simulink model "FM_RDS_Receiver_with_RTL_SDR"  (R2020a)
settings: Solver=FixedStepDiscrete  StartTime=0.0  StopTime=inf  RelTol=1e-3  EnableMultiTasking=on
PreLoadFcn:
  | rds_mf_3;
undefined symbols (not defined in the file or in its folder): dfilt, j
libraries: dsparch4 x5, dspobslib x3, dspsrcs4 x2, commutil2 x1, commsrccod2 x1, dspsigops x1, sdrrlib x1
settings Model: Creator=roppel  LastModifiedBy=roppel
settings DataIOCC: LimitDataPoints=on  SaveFormat=Array  ReturnWorkspaceOutputs=off
settings OptimizationCC: LifeSpan=inf
settings DebuggingCC: SolverPrmCheckMsg=warning  SFUnexpectedBacktrackingDiag=warning  SFNoUnconditionalDefaultTransitionDiag=warning  ArithmeticOperatorsInVariantConditions=warning
settings HardwareCC: ProdBitPerPointer=32  ProdBitPerSizeT=32  ProdBitPerPtrDiffT=32  ProdLargestAtomicFloat=None  ProdIntDivRoundTo=Undefined  ProdEndianess=Unspecified  ProdWordSize=32  ProdHWDeviceType=32-bit Generic
settings ModelReferenceCC: PropagateSignalLabelsOutOfModel=off
settings SFSimCC: SimUseLocalCustomCode=off  CustomCodeUndefinedFunction=UseInterfaceOnly
settings RTWCC: RTWUseLocalCustomCode=off
settings CodeAppCC: StateflowObjectComments=on
settings GRTTargetCC: TargetLangStandard=C89/C90 (ANSI)
settings ConfigComp: CovMetricSettings=dw  CovHtmlReporting=on  CovSaveCumulativeToWorkspaceVar=on  CovSaveSingleToWorkspaceVar=on  CovExternalEMLEnable=off  CovSFcnEnable=off

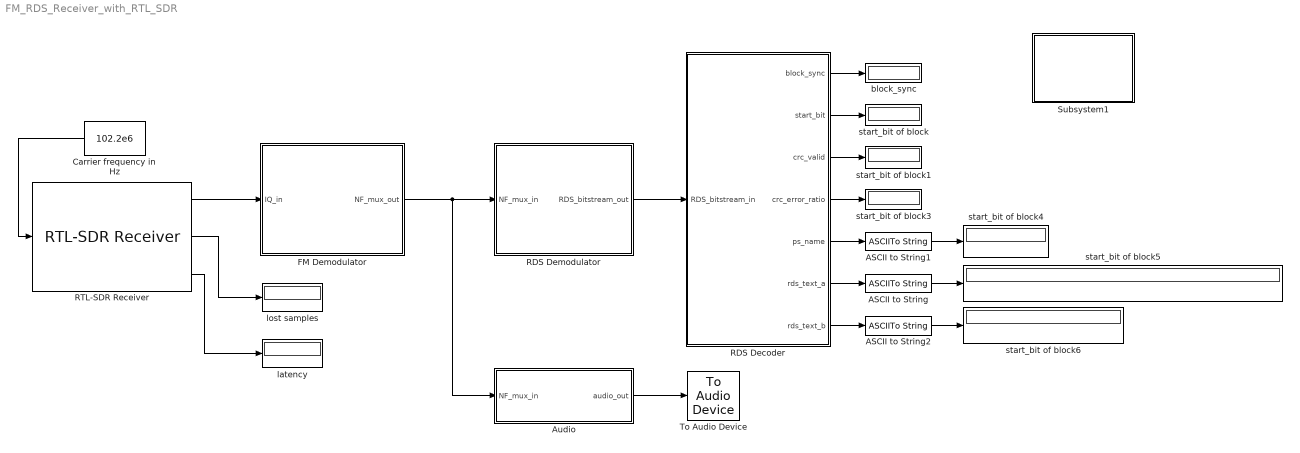
== system FM_RDS_Receiver_with_RTL_SDR ==
  ASCII to String : ASCIIToString
  ASCII to String1 : ASCIIToString
  ASCII to String2 : ASCIIToString
  Audio : Subsystem
  Carrier frequency in Hz : Constant  Value=102.2e6
  FM Demodulator : Subsystem
  RDS Decoder : Subsystem
  RDS Demodulator : Subsystem
  RTL-SDR Receiver : sdrrlib/RTL-SDR Receiver  IPAddress=0  CenterFrequencySource=Input port  CenterFrequency=102.5e6  GainSource=AGC  Gain=50  ADCRate=912e3  FrequencyCorrection=0  LostSamplesOutputPort=on  LatencyOutputPort=on  OutputDataType=single  FrameLength=4864  EnableBurstMode=off  NumFramesInBurst=20  sobjType=sdrr.internal.SDRRTLReceiverSL  dataUDPPort=-1  ctrlUDPPort=-1  subDeviceList=nosubdev  sdrBlockType=SDRBlockTypeSLT.SDRRxBlock  requester=UNUSED_BY_SFCN  sdrExecutionMode=SDRExecutionModeSLT.ExecModeHW  BypassUserLogic=off  DecimatorSelect=DDC decimator  SourceSelect=RF data  SineAmplitude=16000  EnableInternalClock=off  BypassIQBalance=off  IFBandwidth=40e6  ADCRateSource=Dialog  IntermediateFrequency=0  DecimationFactorSource=Dialog  DecimationFactor=512  RFFrequencyIsTunable=logical(1)  SampleTime=(4864)/(912e3)  IFBandwidthSource=Dialog  SineFrequency=30000  BypassDCBlockingFilter=off  IntermediateFrequencySource=Dialog  IQBalanceCoefficients=64  SkipAllHardwareResetAndInitialization=off  EnableIQCalibrationTable=on  CacheIQCalibrationTable=off  EnableOffsetTuning=off  EnableRTLAGC=off  EnableTestMode=off  EnableTunerAGC=on  FrequencyCorrectionSource=Dialog  NumMLBuffers=128  NumUSBBuffers=16  RTLCrystalFrequency=28800000  TunerCrystalFrequency=28800000
      settings: SourceProductBaseCode=RTLSDR
  Subsystem1 : Subsystem  Description=xxx
      settings: OpenFcn=winopen('FM_RDS_Receiver_with_RTL_SDR.pdf')
      mask Display: image('$imagefile'); % Use "Edit Image" on toolstrip to change.
  To Audio Device : dspobslib/To Audio Device  deviceName=Default  inheritSampleRate=on  sampleRate=44100  deviceDatatype=Determine from input data type  autoBufferSize=on  bufferSize=4096  queueDuration=1.0  defaultOutputChannelMapping=on  outputChannelMapping=1  outputNumUnderrunSamples=off
      settings: SourceProductBaseCode=DS
  block_sync : Display
  latency : Display
  lost samples : Display
  start_bit of block{,1,3..6} (6 alike) : Display
  wires:
  RTL-SDR Receiver/1 -> FM Demodulator/1(IQ_in)
  RTL-SDR Receiver/2 -> lost samples/1
  RTL-SDR Receiver/3 -> latency/1
  FM Demodulator/1(NF_mux_out) -> Audio/1(NF_mux_in), RDS Demodulator/1(NF_mux_in)
  Audio/1(audio_out) -> To Audio Device/1
  Carrier frequency in Hz/1 -> RTL-SDR Receiver/1
  RDS Demodulator/1(RDS_bitstream_out) -> RDS Decoder/1(RDS_bitstream_in)
  RDS Decoder/2(start_bit) -> start_bit of block/1
  RDS Decoder/1(block_sync) -> block_sync/1
  RDS Decoder/3(crc_valid) -> start_bit of block1/1
  RDS Decoder/4(crc_error_ratio) -> start_bit of block3/1
  RDS Decoder/6(rds_text_a) -> ASCII to String/1
  ASCII to String/1 -> start_bit of block5/1
  RDS Decoder/5(ps_name) -> ASCII to String1/1
  ASCII to String1/1 -> start_bit of block4/1
  RDS Decoder/7(rds_text_b) -> ASCII to String2/1
  ASCII to String2/1 -> start_bit of block6/1

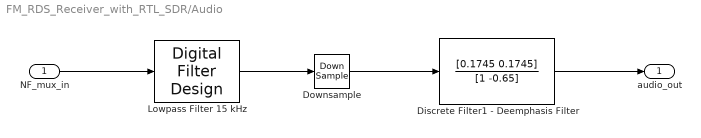
== system FM_RDS_Receiver_with_RTL_SDR/Audio ==
  NF_mux_in : Inport
  Discrete Filter1 - Deemphasis Filter : DiscreteFilter  Numerator=[0.1745 0.1745]  Denominator=[1 -0.65]  InputProcessing=Columns as channels (frame based)  FilterStructure=Direct form I
  Downsample : DownSample  N=19
  Lowpass Filter 15 kHz : dsparch4/Digital Filter Design  mwdsp_browser_bugfix_var=off
  audio_out : Outport
  wires:
  NF_mux_in/1 -> Lowpass Filter 15 kHz/1
  Lowpass Filter 15 kHz/1 -> Downsample/1
  Discrete Filter1 - Deemphasis Filter/1 -> audio_out/1
  Downsample/1 -> Discrete Filter1 - Deemphasis Filter/1

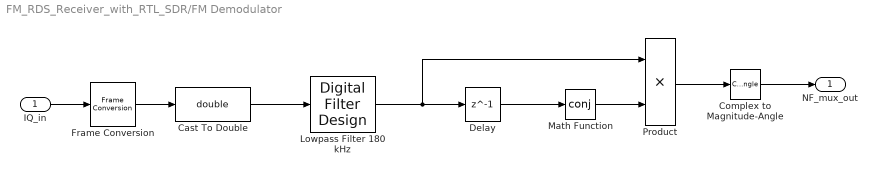
== system FM_RDS_Receiver_with_RTL_SDR/FM Demodulator ==
  IQ_in : Inport
  Cast To Double : DataTypeConversion  OutDataTypeStr=double
  Complex to Magnitude-Angle : ComplexToMagnitudeAngle  Output=Angle
  Delay : Delay  DelayLength=1  InitialCondition=0  InputProcessing=Columns as channels (frame based)
  Frame Conversion : FrameConversion
  Lowpass Filter 180 kHz : dsparch4/Digital Filter Design  mwdsp_browser_bugfix_var=off
  Math Function : Math  Operator=conj  SaturateOnIntegerOverflow=on
  Product : Product
  NF_mux_out : Outport
  wires:
  IQ_in/1 -> Frame Conversion/1
  Product/1 -> Complex to Magnitude-Angle/1
  Math Function/1 -> Product/2
  Delay/1 -> Math Function/1
  Frame Conversion/1 -> Cast To Double/1
  Cast To Double/1 -> Lowpass Filter 180 kHz/1
  Lowpass Filter 180 kHz/1 -> Delay/1, Product/1
  Complex to Magnitude-Angle/1 -> NF_mux_out/1

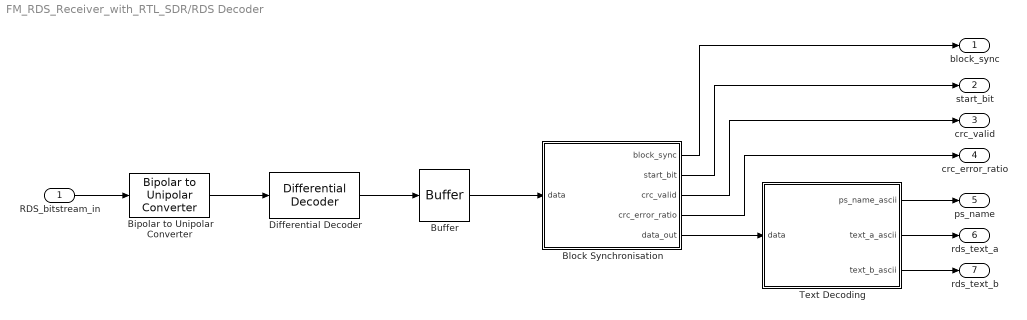
== system FM_RDS_Receiver_with_RTL_SDR/RDS Decoder ==
  RDS_bitstream_in : Inport
  Bipolar to Unipolar Converter : commutil2/Bipolar to Unipolar Converter  M=2  polarity=Positive  dataType=Inherit via internal rule
      settings: SourceProductBaseCode=CM
  Block Synchronisation : MATLAB Function  TreatAsAtomicUnit=on
  Buffer : Buffer  N=10400  V=26
  Differential Decoder : commsrccod2/Differential Decoder  InitCond=0
      settings: SourceProductBaseCode=CM
  Text Decoding : MATLAB Function  TreatAsAtomicUnit=on
  block_sync : Outport
  start_bit : Outport  Port=2
  crc_valid : Outport  Port=3
  crc_error_ratio : Outport  Port=4
  ps_name : Outport  Port=5
  rds_text_a : Outport  Port=6
  rds_text_b : Outport  Port=7
  wires:
  RDS_bitstream_in/1 -> Bipolar to Unipolar Converter/1
  Buffer/1 -> Block Synchronisation/1(data)
  Bipolar to Unipolar Converter/1 -> Differential Decoder/1
  Block Synchronisation/5(data_out) -> Text Decoding/1(data)
  Differential Decoder/1 -> Buffer/1
  Block Synchronisation/1(block_sync) -> block_sync/1
  Block Synchronisation/2(start_bit) -> start_bit/1
  Block Synchronisation/4(crc_error_ratio) -> crc_error_ratio/1
  Text Decoding/1(ps_name_ascii) -> ps_name/1
  Text Decoding/2(text_a_ascii) -> rds_text_a/1
  Text Decoding/3(text_b_ascii) -> rds_text_b/1
  Block Synchronisation/3(crc_valid) -> crc_valid/1

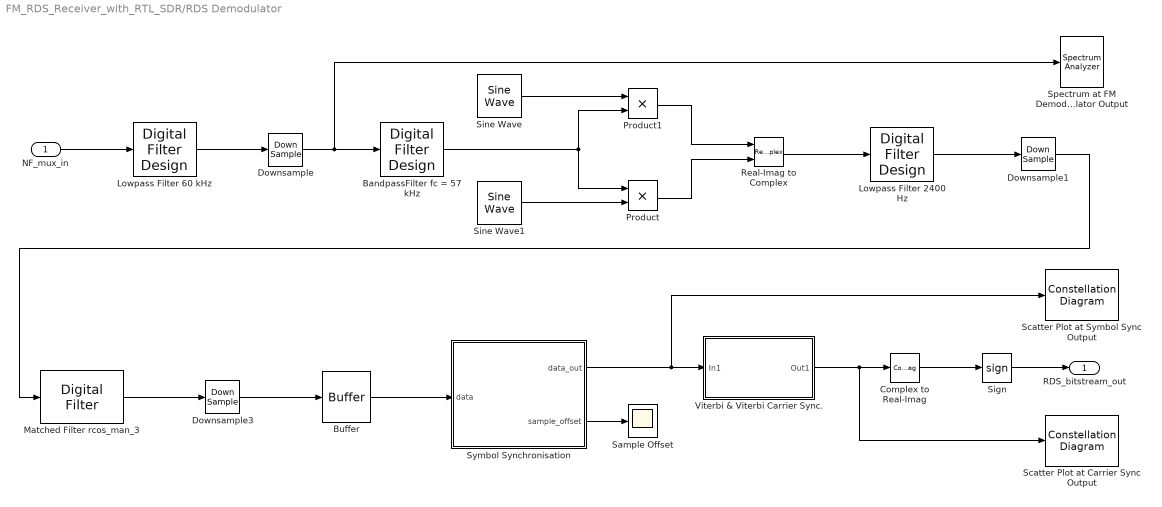
== system FM_RDS_Receiver_with_RTL_SDR/RDS Demodulator ==
  NF_mux_in : Inport
  BandpassFilter fc = 57 kHz : dsparch4/Digital Filter Design  mwdsp_browser_bugfix_var=off
  Buffer : Buffer  N=32*100
  Complex to Real-Imag : ComplexToRealImag  Output=Real
  Downsample : DownSample  N=4  RateOptions=Allow multirate processing
  Downsample1 : DownSample  N=3  RateOptions=Allow multirate processing
  Downsample3 : DownSample  RateOptions=Allow multirate processing
  Lowpass Filter 2400 Hz : dsparch4/Digital Filter Design  mwdsp_browser_bugfix_var=off
  Lowpass Filter 60 kHz : dsparch4/Digital Filter Design  mwdsp_browser_bugfix_var=off
  Matched Filter rcos_man_3 : dspobslib/Digital Filter  TypePopup=FIR (all zeros)  IIRFiltStruct=Direct form II transposed  AllPoleFiltStruct=Direct form  FIRFiltStruct=Direct form  CoeffSource=Specify via dialog  NumCoeffs=rcos_man_3  DenCoeffs=[1 0.1]  BiQuadCoeffs=[1 0.3 0.4 1 0.1 0.2]  LatticeCoeffs=[0.2 0.4]  denIgnore=on  FiltPerSampPopup=One filter per frame  IC=0  ICnum=0  ICden=0  roundingMode=Floor  overflowMode=off  ScaleValues=1  scaleValueFracLength=14  stageInFracLength=15  stageOutFracLength=15  FilterSource=Specify via dialog  dfiltObjectName=dfilt.dffir([1 2 1])  InputProcessing=Columns as channels (frame based)
      settings: SourceProductBaseCode=DS
  Product : Product  RndMeth=Zero  OutDataTypeStr=Inherit: Same as first input
  Product1 : Product  RndMeth=Zero  OutDataTypeStr=Inherit: Same as first input
  Real-Imag to Complex : RealImagToComplex
  Sample Offset : Scope
  Scatter Plot at Carrier Sync Output : ConstellationDiagram
  Scatter Plot at Symbol Sync Output : ConstellationDiagram
  Sign : Signum
  Sine Wave : dspsrcs4/Sine Wave  Amplitude=1  Frequency=57000  Phase=pi/2  SampleMode=Discrete  OutComplex=Real  CompMethod=Table lookup  TableSize=Speed  SampleTime=1/228000  SamplesPerFrame=4864  ResetState=Restart at time zero  OutputFrames=on  dataType=double  wordLen=16  udDataType=sfix(16)  fracBitsMode=Best precision  numFracBits=15  OutDataTypeStr=double  LastOutDataTypeStr=double
  Sine Wave1 : dspsrcs4/Sine Wave  Amplitude=1  Frequency=57000  Phase=-pi  SampleMode=Discrete  OutComplex=Real  CompMethod=Table lookup  TableSize=Speed  SampleTime=1/228000  SamplesPerFrame=4864  ResetState=Restart at time zero  OutputFrames=on  dataType=double  wordLen=16  udDataType=sfix(16)  fracBitsMode=Best precision  numFracBits=15  OutDataTypeStr=double  LastOutDataTypeStr=double
  Spectrum at FM Demodulator Output : SpectrumAnalyzer
  Symbol Synchronisation : MATLAB Function  TreatAsAtomicUnit=on
  Viterbi & Viterbi Carrier Sync. : Subsystem
  RDS_bitstream_out : Outport
  wires:
  Downsample/1 -> BandpassFilter fc = 57 kHz/1, Spectrum at FM Demodulator Output/1
  NF_mux_in/1 -> Lowpass Filter 60 kHz/1
  Lowpass Filter 60 kHz/1 -> Downsample/1
  BandpassFilter fc = 57 kHz/1 -> Product1/2, Product/1
  Sine Wave1/1 -> Product/2
  Product1/1 -> Real-Imag to Complex/1
  Product/1 -> Real-Imag to Complex/2
  Real-Imag to Complex/1 -> Lowpass Filter 2400 Hz/1
  Lowpass Filter 2400 Hz/1 -> Downsample1/1
  Downsample1/1 -> Matched Filter rcos_man_3/1
  Matched Filter rcos_man_3/1 -> Downsample3/1
  Viterbi & Viterbi Carrier Sync./1(Out1) -> Complex to Real-Imag/1, Scatter Plot at Carrier Sync Output/1
  Complex to Real-Imag/1 -> Sign/1
  Sign/1 -> RDS_bitstream_out/1
  Buffer/1 -> Symbol Synchronisation/1(data)
  Downsample3/1 -> Buffer/1
  Sine Wave/1 -> Product1/1
  Symbol Synchronisation/1(data_out) -> Viterbi & Viterbi Carrier Sync./1(In1), Scatter Plot at Symbol Sync Output/1
  Symbol Synchronisation/2(sample_offset) -> Sample Offset/1

== system FM_RDS_Receiver_with_RTL_SDR/Subsystem1 ==

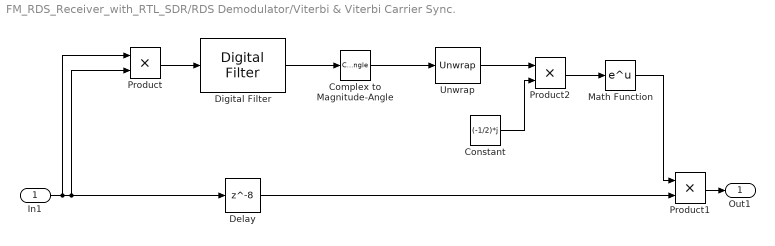
== system FM_RDS_Receiver_with_RTL_SDR/RDS Demodulator/Viterbi & Viterbi Carrier Sync. ==
  In1 : Inport
  Complex to Magnitude-Angle : ComplexToMagnitudeAngle  Output=Angle
  Constant : Constant  Value=(-1/2)*j
  Delay : Delay  DelayLength=8  InitialCondition=0  InputProcessing=Columns as channels (frame based)
  Digital Filter : dspobslib/Digital Filter  TypePopup=FIR (all zeros)  IIRFiltStruct=Direct form II transposed  AllPoleFiltStruct=Direct form  FIRFiltStruct=Direct form  CoeffSource=Specify via dialog  NumCoeffs=ones(1, 17)/17  DenCoeffs=[1 0.1]  BiQuadCoeffs=[1 0.3 0.4 1 0.1 0.2]  LatticeCoeffs=[0.2 0.4]  denIgnore=on  FiltPerSampPopup=One filter per frame  IC=0  ICnum=0  ICden=0  roundingMode=Floor  overflowMode=off  ScaleValues=1  scaleValueFracLength=14  stageInFracLength=15  stageOutFracLength=15  FilterSource=Specify via dialog  dfiltObjectName=dfilt.dffir([1 2 1])  InputProcessing=Columns as channels (frame based)
      settings: SourceProductBaseCode=DS
  Math Function : Math  SignedPower=on  OutputSignalType=complex  SaturateOnIntegerOverflow=on
  Product : Product  RndMeth=Zero
  Product1 : Product  RndMeth=Zero
  Product2 : Product  RndMeth=Zero
  Unwrap : dspsigops/Unwrap  tol=pi  InputProcessing=Columns as channels (frame based)  running=off
  Out1 : Outport
  wires:
  In1/1 -> Product/1, Product/2, Delay/1
  Delay/1 -> Product1/2
  Unwrap/1 -> Product2/1
  Product1/1 -> Out1/1
  Math Function/1 -> Product1/1
  Product/1 -> Digital Filter/1
  Digital Filter/1 -> Complex to Magnitude-Angle/1
  Complex to Magnitude-Angle/1 -> Unwrap/1
  Product2/1 -> Math Function/1
  Constant/1 -> Product2/2

== matlab function FM_RDS_Receiver_with_RTL_SDR/RDS Demodulator/Symbol Synchronisation ==
  data: data_out output; sample_offset output; data input
function [data_out, sample_offset] = fcn(data)
% Carsten Roppel, University of Applied Sciences Schmalkalden
% 02.10.2021

% #codegen

osr = 32;                            % osr samples/bit
nbit = floor(length(data)/osr);      % number of bits
data_out = complex(zeros(nbit, 1));  % output: nbit samples of data
sample_offset = 0;                   % sample offset
max_pwr = 0;                         % maximum power

% downsample data by osr with offset i, calculate power, 
% find offset for maximum power 
for i = 0:(osr-1)
    data_ds = downsample(data, osr, i);
    power = mean(abs(data_ds).^2);
    if power > max_pwr   
        max_pwr = power(1, 1);      
        sample_offset = i;
    end
end

% output: downsampled data using sample_offset
data_ds = downsample(data, osr, sample_offset);
data_ds = data_ds(:, 1);
data_out = data_ds(1:nbit);

end

== matlab function FM_RDS_Receiver_with_RTL_SDR/RDS Decoder/Block Synchronisation ==
  data: block_sync output; start_bit output; crc_valid output; crc_error_ratio output; data input; data_out output
function [block_sync, start_bit, crc_valid, crc_error_ratio, data_out] = fcn(data)
% Carsten Roppel, University of Applied Sciences Schmalkalden
% 02.10.2021

% #codegen

% Requires RDS_offset_word.m

len = 10400;                  % number of bits
nblocks = floor(len/26) - 1;  % number of 26-bit-blocks

% data_out: 399-by-17 matrix
data_out = zeros(nblocks, 17);
block_sync = 0;
next_bit = 1;
start_bit = 1;
offset_word = 0;
crc_errors = 0;
crc_errors_inc = 0;
crc_valid = 0;
crc_error_ratio = 0;

data = data';

while next_bit < len - 25
    % search for valid block
    for i = start_bit:(len-25)
        test = data(i:(i + 25));
        offset_word = RDS_offset_word(test);
        if offset_word ~= 0  % valid block found
            start_bit = i;
            block_sync = 1;
            break;
        else                 % no valid block found
            next_bit = i; 
        end
    end
    
    % extract user data
    if block_sync == 1
        for i = 1:(nblocks - floor(start_bit/26))
            test = data((start_bit + (i - 1)*26):(start_bit + (i - 1)*26 + 25));
            offset_word = RDS_offset_word(test);
            if offset_word == 0
                crc_errors_inc = crc_errors_inc + 1;
                crc_errors = crc_errors + 1;
            else
                crc_errors_inc = 0;
                crc_valid = crc_valid + 1;
            end
            next_bit = start_bit + i*26;
            data_out(i, 1) = offset_word;
            data_out(i, 2:17) = test(1:16);
            % check if 4 consecutive CRC errors
            % if yes, assume loss of sync
            if crc_errors_inc == 4
                block_sync = 0;
                crc_errors_inc = 0;
                start_bit = start_bit + i*26;
                break;
            end
        end
    end
end

crc_error_ratio = crc_errors/(crc_valid + crc_errors);

end

== matlab function FM_RDS_Receiver_with_RTL_SDR/RDS Decoder/Text Decoding ==
  data: data input; ps_name_ascii output; text_a_ascii output; text_b_ascii output
function [ps_name_ascii, text_a_ascii, text_b_ascii] = fcn(data)
% Carsten Roppel, University of Applied Sciences Schmalkalden
% 02.10.2021

% data: 399-by-17 matrix
% Column 1: Block type
%           0: crc_error
%           1: a
%           2: b
%           3: c
%           4: c'
%           5: d
% Columns 2-17: Data bits

btype = data(:, 1);
bdata = data(:, 2:17);
blen = length(bdata);

blockbcount = 0;
% 32 decimal = blank (ASCII)
rds_text_a = zeros(1, 64) + 32;   % Radiotext 64 characters
rds_text_b = zeros(1, 32) + 32;   % Radiotext 32 characters
ps_name = zeros(1, 8) + 32;       % Program Service Name 8 characters

% Search block b
for k = 1:length(btype)
    if btype(k) == 2
        blockbcount = 1;
        % Check group types, see EN50067 Table
        if ~any(xor(bdata(k, (1:5)), [0 0 1 0 0])) 
            % group type 2A -> text in blocks c + d
            % segment address: bits 0 to 3 of block b 
            segment_address = bi2de(flip(bdata(k,(13:16))));
            if (blen >= k + 1 && btype(k+1) == 3)     % check if data contains block c
                char1 = bi2de(flip(bdata(k + 1, (1:8))));
                char2 = bi2de(flip(bdata(k + 1, (9:16))));
                if char1 == 0
                    char1 = 32;
                elseif char2 == 0
                    char2 = 32;
                end                
                rds_text_a(4*segment_address + 1) = char1;
                rds_text_a(4*segment_address + 2) = char2;
            end
            
            if (blen >= k + 2 && btype(k+2) == 5)     % check if data contains block d
                char1 = bi2de(flip(bdata(k + 2, (1:8))));
                char2 = bi2de(flip(bdata(k + 2, (9:16))));
                if char1 == 0
                    char1 = 32;
                elseif char2 == 0
                    char2 = 32;
                end                
                rds_text_a(4*segment_address + 3) = char1;
                rds_text_a(4*segment_address + 4) = char2;
            end
            
        elseif ~any(xor(bdata(k,(1:5)), [0 0 1 0 1]))
            % group type 2B -> text in block d 
            % segment address: bits 0 to 3 of block b 
            segment_address = bi2de(flip(bdata(k,(13:16)))); 
            if (blen >= k + 2 && btype(k+2) == 5)     % check if data contains block d
                char1 = bi2de(flip(bdata(k + 2, (1:8))));
                char2 = bi2de(flip(bdata(k + 2, (9:16))));
                if char1 == 0
                    char1 = 32;
                elseif char2 == 0
                    char2 = 32;
                end                
                rds_text_b(2*segment_address + 1) = char1;
                rds_text_b(2*segment_address + 2) = char2;
            end
            
        elseif ~any(xor(bdata(k,(1:5)), [0 0 0 0 0]))
            % group type = 0A -> ps name in block d
            % segment address: bits 0 to 1 of block b 
            segment_address = bi2de(flip(bdata(k,(15:16))));            
            if (blen >= k + 2 && btype(k+2) == 5)     % check if data contains block d
                char1 = bi2de(flip(bdata(k + 2, (1:8))));
                char2 = bi2de(flip(bdata(k + 2, (9:16))));
                if char1 == 0
                    char1 = 32;
                elseif char2 == 0
                    char2 = 32;
                end                
                ps_name(2*segment_address + 1) = char1;
                ps_name(2*segment_address + 2) = char2;
            end
        end
    end
end

text_a_ascii = uint8(rds_text_a)';
text_b_ascii = uint8(rds_text_b)';
ps_name_ascii = uint8(ps_name)';

end
